simulink model "EthanModel"  (R2019b)
settings: Solver=VariableStepAuto  StartTime=0.0  StopTime=10  RelTol=1e-3
values from neighbouring files (symbols this model uses):
  A = double(round(subs(J_x,   [states, inputs], [trim_state, trim_input])*1000)/1000)    [matlab_init.m]
  A_double = [0 1; 0 0]    [matlab_init.m]
  A_s_double = eval(subs(Ad_double,Ts))    [matlab_init.m]
  A_s_single = eval(subs(Ad_single,Ts))    [matlab_init.m]
  A_single = [0]    [matlab_init.m]
  Aaileron = A(5:8,5:8)    [matlab_init.m]
  Aelevator = A(1:4,1:4)    [matlab_init.m]
  Arudder = A(11:12,11:12)    [matlab_init.m]
  Athrust = A(9:10,9:10)    [matlab_init.m]
  B = B*MotorMix    [matlab_init.m]
  B_double = [0; 1]    [matlab_init.m]
  B_s_double = eval(subs(Bd_double,Ts))    [matlab_init.m]
  B_s_single = eval(subs(Bd_single,Ts))    [matlab_init.m]
  B_single = [1]    [matlab_init.m]
  Baileron = B(5:8,3)    [matlab_init.m]
  Belevator = B(1:4,2)    [matlab_init.m]
  Brudder = B(11:12,4)    [matlab_init.m]
  Bthrust = B(9:10,1)    [matlab_init.m]
  C = double(round(subs(J_y,   [states, inputs], [trim_state, trim_input])*1000)/1000)    [matlab_init.m]
  C_double = [1 0]    [matlab_init.m]
  C_P = 0.041    [matlab_init.m]
  C_rollpitch = rho*prop_dia^4*prop_dist/sqrt(2)*[                 1  -1  -1   1 ;                 1   1  -1  -1 ;                 0   0   0   0 ; ]    [matlab_init.m]
  C_single = [1]    [matlab_init.m]
  C_T = [0.069075;4.95e-05]    [matlab_init.m]
  C_yaw = rho*prop_dia^5/(2*pi)*[                 0   0   0   0 ;                 0   0   0   0 ;                -1   1  -1   1 ; ]    [matlab_init.m]
  Caileron = [0 1 0 0; 0 0 0 1]    [matlab_init.m]
  Celevator = [0 1 0 0; 0 0 0 1]    [matlab_init.m]
  Crudder = [0 1]    [matlab_init.m]
  Cthrust = [ 1 0; 0 0]    [matlab_init.m]
  D = D*MotorMix    [matlab_init.m]
  D_double = [0]    [matlab_init.m]
  D_single = [0]    [matlab_init.m]
  Daileron = [0 ; 0]    [matlab_init.m]
  Delevator = [0 ; 0]    [matlab_init.m]
  Drudder = 0    [matlab_init.m]
  Dthrust = [0 ; D(4,1)]    [matlab_init.m]
  g = [0;0;UAV_mass*9.81]    [matlab_init.m]
  I_flip = eye(12)    [matlab_init.m]
  J = [      Jxx   0   0 ;       0   Jyy  0 ;       0    0  Jzz; ]    [matlab_init.m]
  Jinv = inv(J)    [matlab_init.m]
  L_double = lqe(A_double, G_double, C_double, q_double, r_double, 0)    [matlab_init.m]
  L_single = lqe(A_single, G_single, C_single, q_single, r_single, 0)    [matlab_init.m]
  measurement_noise = 0.1    [matlab_init.m]
  MotorMix = [                 1  1  1 -1 ;                 1  1 -1  1 ;                 1 -1 -1 -1 ;                 1 -1  1  1 ; ]    [matlab_init.m]
  omega_c = 2*pi *20    (= 125.663706144)    [matlab_init.m]
  process_noise = 0.05    [matlab_init.m]
  Prop_H = 2*pi*Jprop*[               0  0  0  0 ;               0  0  0  0 ;               1 -1  1 -1 ; ]    [matlab_init.m]
  q_single = cov(out.In_Out_Data{1}.Values.Data)*10000000000000    [matlab_init.m]
  r_single = cov(out.In_Out_Data{2}.Values.Data)    [matlab_init.m]
  tau2 = 1/(20*pi)    (= 0.0159154943092)    [matlab_init.m]
  Thrust_Sum = rho*prop_dia^4*[                 0   0   0   0 ;                 0   0   0   0 ;                -1  -1  -1  -1 ; ]    [matlab_init.m]
  trim_input = [293,293,293,293]    [matlab_init.m]
  trim_state = [0,0,0,0,0,0,0,0,0,0,0,0]    [matlab_init.m]
  Ts = 0.005    [matlab_init.m]
  UAV_mass = 0.068    [matlab_init.m]
undefined symbols (not defined in the file or in its folder): DiscIntNeverNeededParam, Discrete, Time
libraries: ctrlSharedLib x10, simulink x4, vrlib x3, dspmtrx3 x1
(part 1 of 2)
settings Model: Creator=Chris  LastModifiedBy=ethan

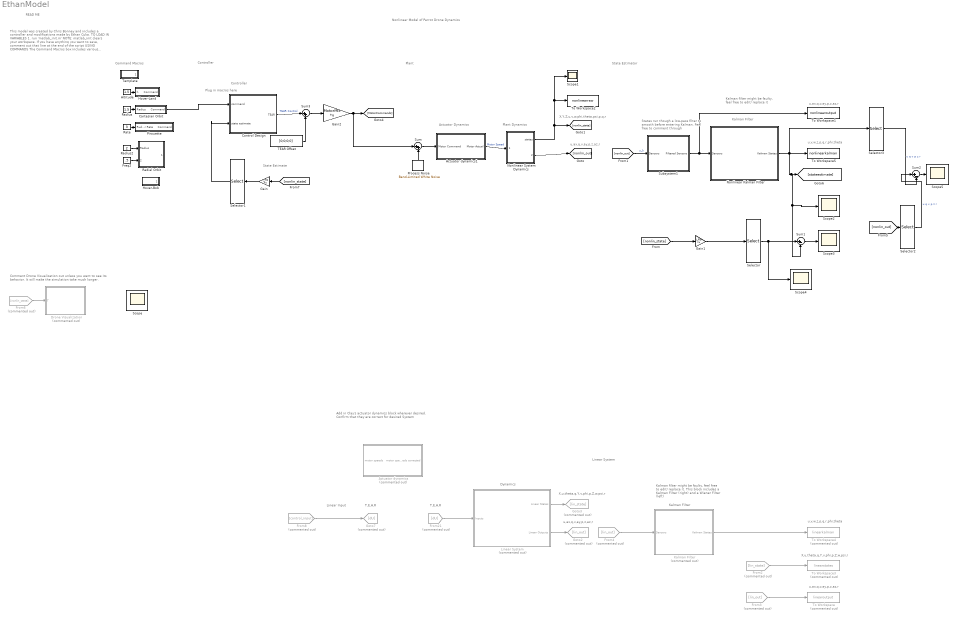
== system EthanModel ==
  note: Plug in macros here
  note: State Estimator
  note: Controller
  note: Command Macros
  note: Add in Clay's actuator dynamics block wherever desired.
      | Confirm that they are correct for desired System
  note: States run though a low-pass filter
      | to smooth before entering Kalman.
      | Feel free to comment through
  note: Kalman filter might be faulty,
      | feel free to edit/ replace it
  note: Comment Drone Visualization out unless you want to see
      | its behavior. It will make the simulation take much longer.
  note: Linear Input
  note: This model was created by Chris Bonney and
      | includes a controller and modifications made
      | by Ethan Cuka.
      |
      |
      | TO LOAD IN VARIABLES
      | 1. run 'matlab_init.m'
      |
      |
      | NOTE: matlab_init clears your workspace.
      | If you have anything you want to save,
      | comment out that line at the end of the script
      |
      |
      | USING COMMANDS
      | The Command Macros box includes various
      | commands to issue to the UAV. To use them,
      | attach their output to the "command" input of
      | the Controller subsystem.
      |
      |
      | READING OUTPUTS
      | most outputs should have a list of variables
      | above them, which are the order they are in
      | for the vector
      |
      |
      | NOISE
      | process and measurement noise blocks are all
      | included in the design, but set to zero power
      | (off); to turn them on go in and adjust their
      | power, there are preset values for noises in
      | kalman_matrices_calculator.m
      |
      |
      | VISUALIZATION
      | 1. the drone visualization block (below) can be
      | uncommented to see the drone fly while
      | running the simulation.
      | 2. I created a scope block (right) that can be
      | copied with preset settings to make viewing
      | data easier
  note: Plant
  note: Kalman Filter
  note: Plant Dynamics
  note: Nonlinear Model of Parrot Drone Dynamics
  note: u,ax,q,v,ay,p,z,az,r
  note: u,v,w,z,p,q,r,phi,theta
  note: Linear System
  note: u,ax,q,v,ay,p,z,az,r
  note: X,u,theta,q,Y,v,phi,p,Z,w,psi,r
  note: u,ax,q,v,ay,p,z,az,r
  note: u,v,w,z,p,q,r,phi,theta
  note: Dynamics
  note: Kalman Filter
  note: Kalman filter might be faulty,
      | feel free to edit/ replace it. This
      | block includes a Kalman Filter (right)
      | and a Wiener Filter (left)
  note: X,Y,Z,u,v,w,phi,theta,psi,p,q,r
  note: u,ax,q,v,ay,p,z,az,r
  note: X,u,theta,q,Y,v,phi,p,Z,w,psi,r
  note: READ ME
  note: T,E,A,R
  note: T,E,A,R
  note: Actuator Dynamics
  note: Controller
  note: State Estimate
  Actuator dynamics : Subsystem  Commented=on
  Actuator dynamics1 : Subsystem
  Altitude : Constant  Value=1.5
  Cartesian Orbit : Subsystem
  Control Design : Subsystem
  Drone Visualization : MATLAB Function  Commented=on  TreatAsAtomicUnit=on
  Freq2 : Constant  Value=.5
  From2 : From  Commented=on  GotoTag=lin_state
  From21 : From  Commented=on  GotoTag=dU
  From3 : From  Commented=on  GotoTag=lin_out
  From4 : From  Commented=on  GotoTag=lin_out
  From6 : From  Commented=on  GotoTag=nonlin_state
  From8 : From  Commented=on  GotoTag=control_input
  Gain : Gain  Gain=I_flip  Multiplication=Matrix(K*u)
  Gain1 : Gain  Gain=I_flip  Multiplication=Matrix(K*u)
  Gain2 : Gain  Gain=MotorMix  Multiplication=Matrix(K*u)
      settings: AttributesFormatString=%<Gain>
  Goto2 : Goto  Commented=on  GotoTag=lin_out
  Goto3 : Goto  Commented=on  GotoTag=lin_state
  Goto7 : Goto  Commented=on  GotoTag=dU
  Hover-Bob : Subsystem
  Hover-Land : Subsystem
  Kalman Filter : Subsystem  Commented=on
  Linear System : Subsystem  Commented=on
  Nonlinear Kalman Filter : Subsystem
  Nonlinear System Dynamics : Subsystem
  Pirouette : Subsystem
  Process Noise : simulink/Sources/Band-Limited White Noise  Cov=process_noise*ones(4,1)*0  Ts=0.05  seed=[1;2;3;4]
  Radial Orbit : Subsystem
  Radius : Constant  Value=1.5
  Radius2 : Constant  Value=2
  Rate : Constant  Value=3
  Scope{,1..5} (6 alike) : Scope
  Selector : Selector  InputPortWidth=12  IndexOptions=Index vector (dialog)  Indices=[4 5 6 3 10 11 12 7 8]  OutputSizes=1
  Selector1 : Selector  InputPortWidth=12  IndexOptions=Index vector (dialog)  Indices=[4 5 6 3 10 11 12 7 8]  OutputSizes=1
  Selector2 : Selector  InputPortWidth=9  IndexOptions=Index vector (dialog)  Indices=[1 3 4 6 7 9]  OutputSizes=1
  Selector3 : Selector  InputPortWidth=9  IndexOptions=Index vector (dialog)  Indices=[1 6 2 5 4 7]  OutputSizes=1
  Subsystem1 : Subsystem
  Sum : Sum  Inputs=|++
  Sum1 : Sum  Inputs=|+-
  Sum2 : Sum  Inputs=|+-
  Sum3 : Sum  Inputs=|++
  TEAR Offset : Constant  Value=[0;0;0;0]
  Template : Subsystem
  To Workspace : ToWorkspace  Commented=on  VariableName=linearoutput  SaveFormat=Timeseries  SampleTime=-1
  To Workspace1 : ToWorkspace  VariableName=nonlinearoutput  SaveFormat=Timeseries  SampleTime=-1
  To Workspace2 : ToWorkspace  VariableName=nonlinearraw  SampleTime=-1
  To Workspace3 : ToWorkspace  Commented=on  VariableName=linearstates  SaveFormat=Timeseries  SampleTime=-1
  To Workspace4 : ToWorkspace  Commented=on  VariableName=linearkalman  SaveFormat=Timeseries  SampleTime=-1
  To Workspace5 : ToWorkspace  VariableName=nonlinearkalman  SaveFormat=Timeseries  SampleTime=-1
  wires:
  From4/1 -> Kalman Filter/1(Sensors)
  From8/1 -> Goto7/1
  From3/1 -> To Workspace/1
  From2/1 -> To Workspace3/1
  Subsystem1/1(Filtered Sensors) -> Nonlinear Kalman Filter/1(Sensors), To Workspace1/1
  Linear System/1(Linear States) -> Goto3/1
  Nonlinear Kalman Filter/1(Kalman States) -> Selector3/1, Scope2/1, Sum1/2, [stateestimate], To Workspace5/1
  From21/1 -> Linear System/1("Inputs ")
  Actuator dynamics1/1(Motor Actual) -> Nonlinear System Dynamics/1(inputs n)  "Motor Speed"
  Nonlinear System Dynamics/1(states) -> Scope1/1, To Workspace2/1, [nonlin_state]
  Linear System/2(Linear Outputs) -> Goto2/1
  [nonlin_out] -> Subsystem1/1(Sensors)  "y_k"
  Nonlinear System Dynamics/2(outputs) -> [nonlin_out]
  Kalman Filter/1(Kalman States) -> To Workspace4/1
  From6/1 -> Drone Visualization/1(T)
  Gain2/1 -> Sum/1, [MotorCommands]
  Sum/1 -> Actuator dynamics1/1(Motor Command)
  Process Noise/1 -> Sum/2
  [nonlin_state] -> Gain1/1
  Sum1/1 -> Scope3/1
  [nonlin_state] -> Gain/1
  Gain/1 -> Selector1/1
  Selector/1 -> Scope4/1, Sum1/1
  Radius/1 -> Cartesian Orbit/1(Radius)
  Altitude/1 -> Hover-Land/1(h)
  Gain1/1 -> Selector/1
  Sum2/1 -> Scope5/1
  Selector2/1 -> Sum2/1  "u q v p z r"
  Selector3/1 -> Sum2/2  "u q v p z r"
  [nonlin_out] -> Selector2/1
  Control Design/1(TEAR) -> Sum3/1  "TEAR Control"
  Sum3/1 -> Gain2/1
  TEAR Offset/1 -> Sum3/2
  Selector1/1 -> Control Design/2(state estimate)
  Rate/1 -> Pirouette/1(Rudder Rate)
  Freq2/1 -> Radial Orbit/2(Frequency)
  Radius2/1 -> Radial Orbit/1("Radius ")
  Cartesian Orbit/1(Command) -> Control Design/1(command)

== system EthanModel/Actuator dynamics ==
  note: Ignoring Gain V/V0 because
      | we can correct for it
  motor speeds : Inport
  30ms delay : TransportDelay  DelayTime=30e-3
  Demux : Demux
  Mux : Mux
  Saturation4 : Saturate  UpperLimit=500  LowerLimit=10
  Sum2 : Sum  Inputs=++|
  Transfer Fcn : TransferFcn  Denominator=[tau2 1]
  Transfer Fcn1 : TransferFcn  Denominator=[tau2 1]
  Transfer Fcn2 : TransferFcn  Denominator=[tau2 1]
  actuator transfer function : TransferFcn  Denominator=[tau2 1]
  speed correction : Constant  Value=trim_input(1)
  motor speeds corrected : Outport
  wires:
  speed correction/1 -> Sum2/1
  Sum2/1 -> Saturation4/1
  Demux/2 -> Transfer Fcn1/1
  30ms delay/1 -> Demux/1
  Demux/4 -> actuator transfer function/1
  Demux/1 -> Transfer Fcn/1
  Demux/3 -> Transfer Fcn2/1
  motor speeds/1 -> 30ms delay/1
  Saturation4/1 -> motor speeds corrected/1
  Transfer Fcn/1 -> Mux/1
  Transfer Fcn1/1 -> Mux/2
  Transfer Fcn2/1 -> Mux/3
  actuator transfer function/1 -> Mux/4
  Mux/1 -> Sum2/2

== system EthanModel/Actuator dynamics1 ==
  note: Ignoring Gain V/V0 because
      | we can correct for it
  Motor Command : Inport
  30ms delay : TransportDelay  DelayTime=30e-3
  Constant2 : Constant  Value=trim_input'  VectorParams1D=off
  Demux : Demux
  Mux : Mux
  Saturation4 : Saturate  UpperLimit=500  LowerLimit=10
  Scope : Scope
  Sum2 : Sum  Inputs=++|
  Transfer Fcn : TransferFcn  Denominator=[tau2 1]
  Transfer Fcn1 : TransferFcn  Denominator=[tau2 1]
  Transfer Fcn2 : TransferFcn  Denominator=[tau2 1]
  actuator transfer function : TransferFcn  Denominator=[tau2 1]
  Motor Actual : Outport
  wires:
  Mux/1 -> Sum2/2
  actuator transfer function/1 -> Mux/4
  Transfer Fcn2/1 -> Mux/3
  Transfer Fcn1/1 -> Mux/2
  Transfer Fcn/1 -> Mux/1
  Saturation4/1 -> Scope/1, Motor Actual/1
  Motor Command/1 -> 30ms delay/1
  Demux/3 -> Transfer Fcn2/1
  Demux/1 -> Transfer Fcn/1
  Demux/4 -> actuator transfer function/1
  30ms delay/1 -> Demux/1
  Demux/2 -> Transfer Fcn1/1
  Sum2/1 -> Saturation4/1
  Constant2/1 -> Sum2/1

== system EthanModel/Cartesian Orbit ==
  note: This command macro causes the drone to orbit by giving it a sinusoidal command to the x and y velocities
  Radius : Inport
  Gain : Gain  Gain=1/(2*pi)
  Mux1 : Mux  Inputs=9
  Product : Product  Inputs=3
  Product1 : Product  Inputs=3
  Sine Wave : Sin  Amplitude=3  Phase=-1  SampleTime=0
  Sine Wave1 : Sin  Amplitude=3  Phase=pi/2-1  SampleTime=0
  Step : Step  SampleTime=0
  Step1 : Step  SampleTime=0
  height1 : Constant  Value=1.5
  p1 : Constant  Value=0
  phi1 : Constant  Value=0
  q1 : Constant  Value=0
  r1 : Constant  Value=0
  theta1 : Constant  Value=0
  w1 : Constant  Value=0
  Command : Outport
  wires:
  Product1/1 -> Mux1/2
  Step1/1 -> Product1/1
  Sine Wave1/1 -> Product1/2
  Step/1 -> Product/2
  Sine Wave/1 -> Product/1
  Product/1 -> Mux1/1
  Mux1/1 -> Command/1
  phi1/1 -> Mux1/9
  q1/1 -> Mux1/6
  height1/1 -> Mux1/4
  w1/1 -> Mux1/3
  theta1/1 -> Mux1/8
  p1/1 -> Mux1/5
  r1/1 -> Mux1/7
  Radius/1 -> Gain/1
  Gain/1 -> Product1/3, Product/3

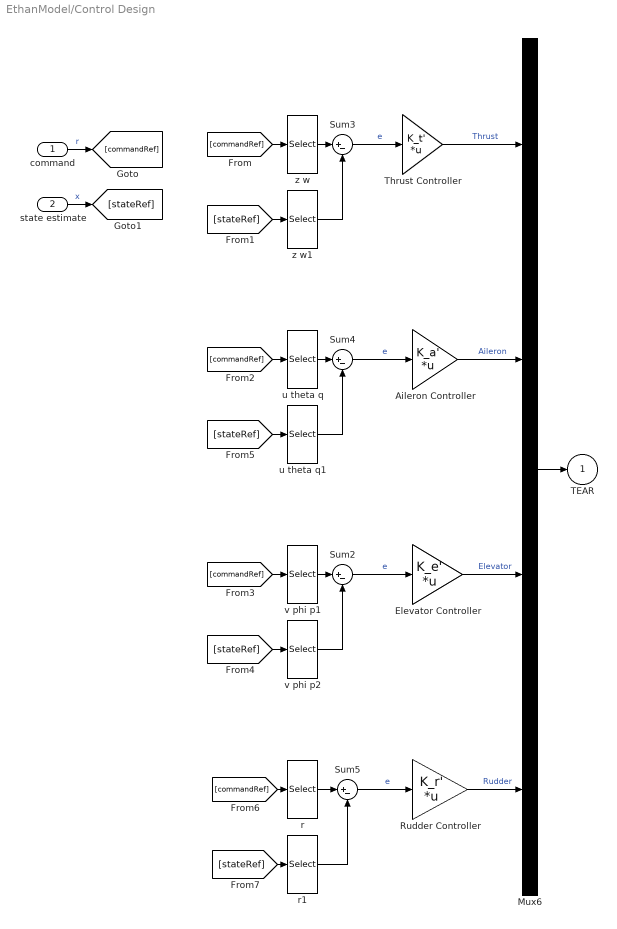
== system EthanModel/Control Design ==
  command : Inport
  state estimate : Inport  Port=2
  Aileron Controller : Gain  Gain=K_a'  Multiplication=Matrix(K*u)
  Elevator Controller : Gain  Gain=K_e'  Multiplication=Matrix(K*u)
  Mux6 : Mux
  Rudder Controller : Gain  Gain=K_r'  Multiplication=Matrix(K*u)
  Sum{2..5} (4 alike) : Sum  Inputs=|+-
  Thrust Controller : Gain  Gain=K_t'  Multiplication=Matrix(K*u)
  r : Selector  InputPortWidth=9  IndexOptions=Index vector (dialog)  Indices=[7]  OutputSizes=1
  r1 : Selector  InputPortWidth=9  IndexOptions=Index vector (dialog)  Indices=[7]  OutputSizes=1
  u theta q : Selector  InputPortWidth=9  IndexOptions=Index vector (dialog)  Indices=[1 9 6]  OutputSizes=1
  u theta q1 : Selector  InputPortWidth=9  IndexOptions=Index vector (dialog)  Indices=[1 9 6]  OutputSizes=1
  v phi p1 : Selector  InputPortWidth=9  IndexOptions=Index vector (dialog)  Indices=[2 8 5]  OutputSizes=1
  v phi p2 : Selector  InputPortWidth=9  IndexOptions=Index vector (dialog)  Indices=[2 8 5]  OutputSizes=1
  z w : Selector  InputPortWidth=9  IndexOptions=Index vector (dialog)  Indices=[4 3]  OutputSizes=1
  z w1 : Selector  InputPortWidth=9  IndexOptions=Index vector (dialog)  Indices=[4 3]  OutputSizes=1
  TEAR : Outport
  wires:
  Mux6/1 -> TEAR/1
  command/1 -> [commandRef]  "r"
  state estimate/1 -> [stateRef]  "x"
  [commandRef] -> z w/1
  [stateRef] -> z w1/1
  z w/1 -> Sum3/1
  z w1/1 -> Sum3/2
  Sum3/1 -> Thrust Controller/1  "e"
  Thrust Controller/1 -> Mux6/1  "Thrust"
  [stateRef] -> v phi p2/1
  v phi p2/1 -> Sum2/2
  [commandRef] -> v phi p1/1
  v phi p1/1 -> Sum2/1
  u theta q/1 -> Sum4/1
  [commandRef] -> u theta q/1
  u theta q1/1 -> Sum4/2
  Sum4/1 -> Aileron Controller/1  "e"
  [stateRef] -> u theta q1/1
  [commandRef] -> r/1
  [stateRef] -> r1/1
  r/1 -> Sum5/1
  r1/1 -> Sum5/2
  Sum2/1 -> Elevator Controller/1  "e"
  Sum5/1 -> Rudder Controller/1  "e"
  Rudder Controller/1 -> Mux6/4  "Rudder"
  Aileron Controller/1 -> Mux6/2  "Aileron"
  Elevator Controller/1 -> Mux6/3  "Elevator"

== system EthanModel/Hover-Bob ==
  note: This command macro causes the drone to hover up and down by commanding the altitude to follow a square wave with DC offset
  Constant : Constant  Value=.5
  Mux : Mux  Inputs=9
  Pulse Generator : DiscretePulseGenerator  PulseType=Time based  Amplitude=1.5  Period=3  PulseWidth=50
  Sum : Sum  Inputs=|++
  p : Constant  Value=0
  phi : Constant  Value=0
  q : Constant  Value=0
  r : Constant  Value=0
  theta : Constant  Value=0
  u : Constant  Value=0
  v : Constant  Value=0
  w : Constant  Value=0
  Command : Outport
  wires:
  r/1 -> Mux/7
  w/1 -> Mux/3
  phi/1 -> Mux/9
  v/1 -> Mux/2
  q/1 -> Mux/6
  u/1 -> Mux/1
  p/1 -> Mux/5
  theta/1 -> Mux/8
  Mux/1 -> Command/1
  Constant/1 -> Sum/2
  Pulse Generator/1 -> Sum/1
  Sum/1 -> Mux/4

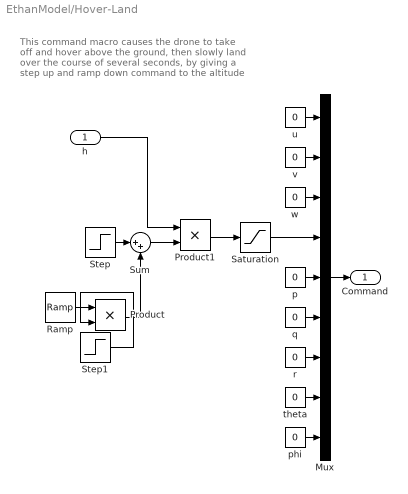
== system EthanModel/Hover-Land ==
  note: This command macro causes the drone to take off and hover above the ground, then slowly land over the course of several seconds, by giving a step up and ramp down command to the altitude
  h : Inport
  Mux : Mux  Inputs=9
  Product : Product
  Product1 : Product
  Ramp : simulink/Sources/Ramp  slope=-.5  start=0  InitialOutput=3.5
  Saturation : Saturate  UpperLimit=100  LowerLimit=0
  Step : Step  SampleTime=0
  Step1 : Step  Time=7  SampleTime=0
  Sum : Sum  Inputs=|++
  p : Constant  Value=0
  phi : Constant  Value=0
  q : Constant  Value=0
  r : Constant  Value=0
  theta : Constant  Value=0
  u : Constant  Value=0
  v : Constant  Value=0
  w : Constant  Value=0
  Command : Outport
  wires:
  Mux/1 -> Command/1
  theta/1 -> Mux/8
  p/1 -> Mux/5
  Product1/1 -> Saturation/1
  u/1 -> Mux/1
  q/1 -> Mux/6
  v/1 -> Mux/2
  phi/1 -> Mux/9
  w/1 -> Mux/3
  r/1 -> Mux/7
  Step/1 -> Sum/1
  Sum/1 -> Product1/2
  Ramp/1 -> Product/1
  Step1/1 -> Product/2
  Product/1 -> Sum/2
  Saturation/1 -> Mux/4
  h/1 -> Product1/1

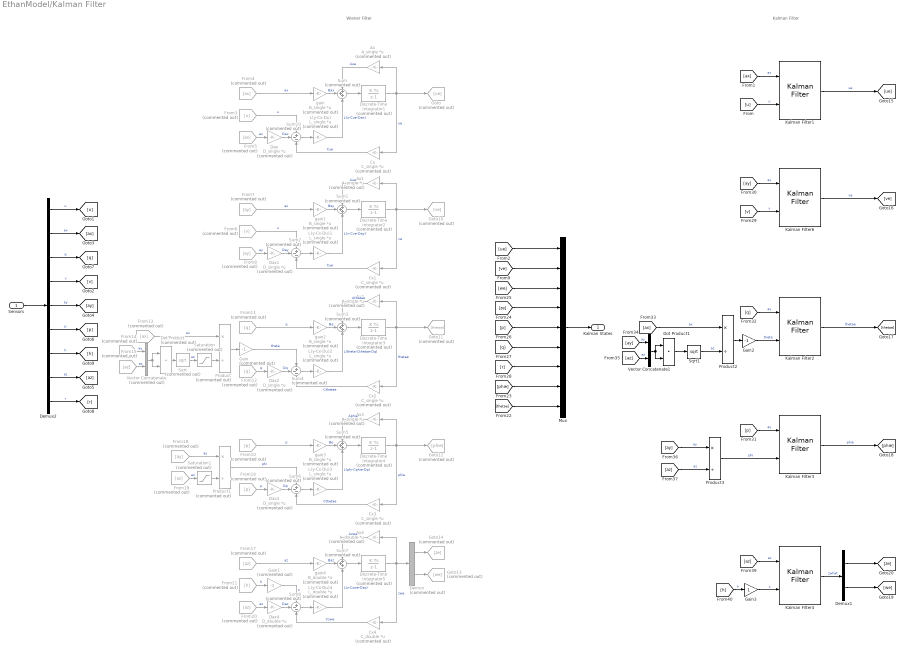
== system EthanModel/Kalman Filter ==
  note: Wiener Filter
  note: Kalman Filter
  Sensors : Inport
  Ax{,1..3} (4 alike) : Gain  Commented=on  Gain=A_single  Multiplication=Matrix(K*u)
      settings: AttributesFormatString=Ax
  Ax4 : Gain  Commented=on  Gain=A_double  Multiplication=Matrix(K*u)
      settings: AttributesFormatString=Ax
  Cx{,1..3} (4 alike) : Gain  Commented=on  Gain=C_single  Multiplication=Matrix(K*u)
      settings: AttributesFormatString=Cx
  Cx4 : Gain  Commented=on  Gain=C_double  Multiplication=Matrix(K*u)
      settings: AttributesFormatString=Cx
  Dax{,1..3} (4 alike) : Gain  Commented=on  Gain=D_single  Multiplication=Matrix(K*u)
      settings: AttributesFormatString=Du
  Dax4 : Gain  Commented=on  Gain=D_double  Multiplication=Matrix(K*u)
      settings: AttributesFormatString=Du
  Demux : Demux  Commented=on  Outputs=2
  Demux1 : Demux  Outputs=2
  Demux2 : Demux  Outputs=9
  Discrete-Time Integrator{1..5} (5 alike) : DiscreteIntegrator  Commented=on  SampleTime=-1  ICPrevOutput=DiscIntNeverNeededParam  ICPrevScaledInput=DiscIntNeverNeededParam
  Dot Product : DotProduct  Commented=on  OutMin=0.0001  InputSameDT=on  OutDataTypeStr=Inherit: Inherit via internal rule
  Dot Product1 : DotProduct  OutMin=0.0001  InputSameDT=on  OutDataTypeStr=Inherit: Inherit via internal rule
  From10 : From  Commented=on  GotoTag=p
  From11 : From  Commented=on  GotoTag=q
  From12 : From  Commented=on  GotoTag=q
  From13 : From  Commented=on  GotoTag=ax
  From{7..8,14,18} (4 alike) : From  Commented=on  GotoTag=ay
  From{15,17,19..20} (4 alike) : From  Commented=on  GotoTag=az
  From16 : From  Commented=on  GotoTag=p
  From21 : From  Commented=on  GotoTag=h
  From3 : From  Commented=on  GotoTag=u
  From4 : From  Commented=on  GotoTag=ax
  From5 : From  Commented=on  GotoTag=ax
  From6 : From  Commented=on  GotoTag=v
  Gain : Gain  Commented=on  Gain=-1
  Gain1 : Gain  Commented=on  Gain=-1
  Gain2 : Gain  Gain=-1
  Gain3 : Gain
  Goto : Goto  Commented=on  GotoTag=ue
  Goto10 : Goto  Commented=on  GotoTag=ve
  Goto11 : Goto  Commented=on  GotoTag=thetae
  Goto12 : Goto  Commented=on  GotoTag=phie
  Goto13 : Goto  Commented=on  GotoTag=we
  Goto14 : Goto  Commented=on  GotoTag=ze
  Kalman Filter{1..3,6} (4 alike) : ctrlSharedLib/Kalman Filter  TimeDomain=Discrete-Time  UseCurrentEstimator=on  ModelSource=Individual A, B, C, D matrices  ModelSourceVariable=ss(0.95,1,1,0,1)  A=A_s_single  B=B_s_single  C=C_single  D=D_single  NumberOfStates=1  NumberOfInputs=1  NumberOfOutputs=1  InitialEstimateSource=Dialog  X0=[0]  P0=10  UseK=off  UseGH=off  NumberOfProcessNoiseInputs=1  G=1  TimeInvariantG=on  H=0  TimeInvariantH=on  Q=[1]*q_single  TimeInvariantQ=on  R=[1]*r_single  TimeInvariantR=on  N=0  TimeInvariantN=on  AddInputPort=on  AddEnablePort=off  OutputEstimatedY=off  OutputP=off  Ts=Ts
      settings: SourceProductBaseCode=CT
  Kalman Filter4 : ctrlSharedLib/Kalman Filter  TimeDomain=Discrete-Time  UseCurrentEstimator=on  ModelSource=Individual A, B, C, D matrices  ModelSourceVariable=ss(0.95,1,1,0,1)  A=A_s_double  B=B_s_double  C=C_double  D=D_double  NumberOfStates=1  NumberOfInputs=1  NumberOfOutputs=1  InitialEstimateSource=Dialog  X0=[0]  P0=10  UseK=off  UseGH=off  NumberOfProcessNoiseInputs=1  G=1  TimeInvariantG=on  H=0  TimeInvariantH=on  Q=[0 0 ; 0 1]*q_single  TimeInvariantQ=on  R=[1]*r_single  TimeInvariantR=on  N=0  TimeInvariantN=on  AddInputPort=on  AddEnablePort=off  OutputEstimatedY=off  OutputP=off  Ts=Ts
      settings: SourceProductBaseCode=CT
  L(y-Cx-Du){,1..3} (4 alike) : Gain  Commented=on  Gain=L_single  Multiplication=Matrix(K*u)
      settings: AttributesFormatString=L(y-Cx-Du)
  L(y-Cx-Du)4 : Gain  Commented=on  Gain=L_double  Multiplication=Matrix(K*u)
      settings: AttributesFormatString=L(y-Cx-Du)
  Mux : Mux  Inputs=9
  Product : Product  Commented=on  Inputs=*/
  Product1 : Product  Commented=on  Inputs=*/
  Product2 : Product  Inputs=*/
  Product3 : Product  Inputs=*/
  Saturation : Saturate  Commented=on  UpperLimit=inf  LowerLimit=0.001
  Saturation1 : Saturate  Commented=on  UpperLimit=inf  LowerLimit=0.001
  Sqrt : Sqrt  Commented=on  SaturateOnIntegerOverflow=on
  Sqrt1 : Sqrt  SaturateOnIntegerOverflow=on
  Sum{,1,3,5,7} (5 alike) : Sum  Commented=on  Inputs=+++
  Sum{2,4,6,8,10} (5 alike) : Sum  Commented=on  Inputs=+--
  Vector Concatenate : Concatenate  Commented=on
  Vector Concatenate1 : Concatenate
  gain{,1..3} (4 alike) : Gain  Commented=on  Gain=B_single  Multiplication=Matrix(K*u)
      settings: AttributesFormatString=Bu
  gain4 : Gain  Commented=on  Gain=B_double  Multiplication=Matrix(K*u)
      settings: AttributesFormatString=Bu
  Kalman States : Outport
  wires:
  Discrete-Time Integrator1/1 -> Goto/1, Cx/1, Ax/1  "ue"
  Sum10/1 -> L(y-Cx-Du)/1
  Ax/1 -> Sum/1  "Aue"
  L(y-Cx-Du)/1 -> Sum/3  "L(u-Cue-Dax)"
  Cx/1 -> Sum10/3  "Cue"
  From4/1 -> gain/1  "ax"
  gain/1 -> Sum/2  "Bax"
  From3/1 -> Sum10/1  "u"
  From5/1 -> Dax/1  "ax"
  Dax/1 -> Sum10/2  "Dax"
  Sum/1 -> Discrete-Time Integrator1/1
  Demux2/1 -> [u]  "u"
  Sensors/1 -> Demux2/1
  Demux2/6 -> [p]  "p"
  Sum1/1 -> Discrete-Time Integrator2/1
  Dax1/1 -> Sum2/2  "Day"
  From8/1 -> Dax1/1  "ay"
  From6/1 -> Sum2/1  "u"
  gain1/1 -> Sum1/2  "Bay"
  From7/1 -> gain1/1  "ax"
  Cx1/1 -> Sum2/3  "Cue"
  L(y-Cx-Du)1/1 -> Sum1/3  "L(v-Cve-Day)"
  Ax1/1 -> Sum1/1  "Aue"
  Sum2/1 -> L(y-Cx-Du)1/1
  Discrete-Time Integrator2/1 -> Ax1/1, Cx1/1, Goto10/1  "ve"
  Discrete-Time Integrator3/1 -> Goto11/1, Cx2/1, Ax2/1  "thetae"
  Sum4/1 -> L(y-Cx-Du)2/1
  Ax2/1 -> Sum3/1  "Athetae"
  L(y-Cx-Du)2/1 -> Sum3/3  "L(theta-Cthetae-Dq)"
  Cx2/1 -> Sum4/3  "Cthetae"
  From11/1 -> gain2/1  "q"
  gain2/1 -> Sum3/2  "Bq"
  Gain/1 -> Sum4/1  "theta"
  From12/1 -> Dax2/1  "q"
  Dax2/1 -> Sum4/2  "Dq"
  Sum3/1 -> Discrete-Time Integrator3/1
  From14/1 -> Vector Concatenate/1  "ay"
  From15/1 -> Vector Concatenate/2  "az"
  Vector Concatenate/1 -> Dot Product/1, Dot Product/2
  Dot Product/1 -> Sqrt/1
  From13/1 -> Product/1  "ax"
  Product/1 -> Gain/1
  From18/1 -> Product1/1  "ay"
  Sum5/1 -> Discrete-Time Integrator4/1
  Dax3/1 -> Sum6/2  "Dp"
  From16/1 -> Dax3/1  "p"
  Product1/1 -> Sum6/1  "phi"
  gain3/1 -> Sum5/2  "Bp"
  From10/1 -> gain3/1  "p"
  Cx3/1 -> Sum6/3  "Cthetae"
  L(y-Cx-Du)3/1 -> Sum5/3  "L(phi-Cphie-Dp)"
  Ax3/1 -> Sum5/1  "Aphie"
  Sum6/1 -> L(y-Cx-Du)3/1
  Discrete-Time Integrator4/1 -> Ax3/1, Cx3/1, Goto12/1  "phie"
  Discrete-Time Integrator5/1 -> Ax4/1, Demux/1, Cx4/1  "zwe"
  Sum8/1 -> L(y-Cx-Du)4/1
  Ax4/1 -> Sum7/1  "Azwe"
  L(y-Cx-Du)4/1 -> Sum7/3  "L(z-Czwe-Daz)"
  Cx4/1 -> Sum8/3  "Czwe"
  From17/1 -> gain4/1  "az"
  gain4/1 -> Sum7/2  "Baz"
  From21/1 -> Gain1/1  "h"
  From20/1 -> Dax4/1  "az"
  Dax4/1 -> Sum8/2  "Daz"
  Sum7/1 -> Discrete-Time Integrator5/1
  Demux/2 -> Goto13/1
  Demux/1 -> Goto14/1
  Gain1/1 -> Sum8/1  "z"
  [ue] -> Mux/1
  [ve] -> Mux/2
  [we] -> Mux/3
  [ze] -> Mux/4
  Mux/1 -> Kalman States/1
  [r] -> Mux/7
  [q] -> Mux/6
  [p] -> Mux/5
  [phie] -> Mux/8
  [thetae] -> Mux/9
  [ax] -> Kalman Filter1/1  "ax"
  [u] -> Kalman Filter1/2  "u"
  [v] -> Kalman Filter6/2  "v"
  [ay] -> Kalman Filter6/1  "ay"
  [q] -> Kalman Filter2/1  "ay"
  Gain2/1 -> Kalman Filter2/2  "theta"
  Sqrt/1 -> Saturation/1  "az"
  Saturation/1 -> Product/2
  From19/1 -> Saturation1/1  "az"
  Saturation1/1 -> Product1/2
  Sqrt1/1 -> Product2/2  "az"
  Product2/1 -> Gain2/1
  [ax] -> Product2/1  "ax"
  Dot Product1/1 -> Sqrt1/1
  Vector Concatenate1/1 -> Dot Product1/2, Dot Product1/1
  [az] -> Vector Concatenate1/2  "az"
  [ay] -> Vector Concatenate1/1  "ay"
  [p] -> Kalman Filter3/1  "ay"
  [az] -> Product3/2  "az"
  Product3/1 -> Kalman Filter3/2  "phi"
  [ay] -> Product3/1  "ay"
  Kalman Filter4/1 -> Demux1/1  "zwhat"
  [az] -> Kalman Filter4/1  "az"
  Gain3/1 -> Kalman Filter4/2  "z"
  Demux1/1 -> [ze]
  Demux1/2 -> [we]
  Kalman Filter3/1 -> [phie]  "phie"
  Kalman Filter2/1 -> [thetae]  "thetae"
  Kalman Filter6/1 -> [ve]  "ve"
  Kalman Filter1/1 -> [ue]  "ue"
  [h] -> Gain3/1  "h"
  Demux2/2 -> [ax]  "ax"
  Demux2/4 -> [v]  "v"
  Demux2/3 -> [q]  "q"
  Demux2/8 -> [az]  "az"
  Demux2/5 -> [ay]  "ay"
  Demux2/7 -> [h]  "h"
  Demux2/9 -> [r]  "r"

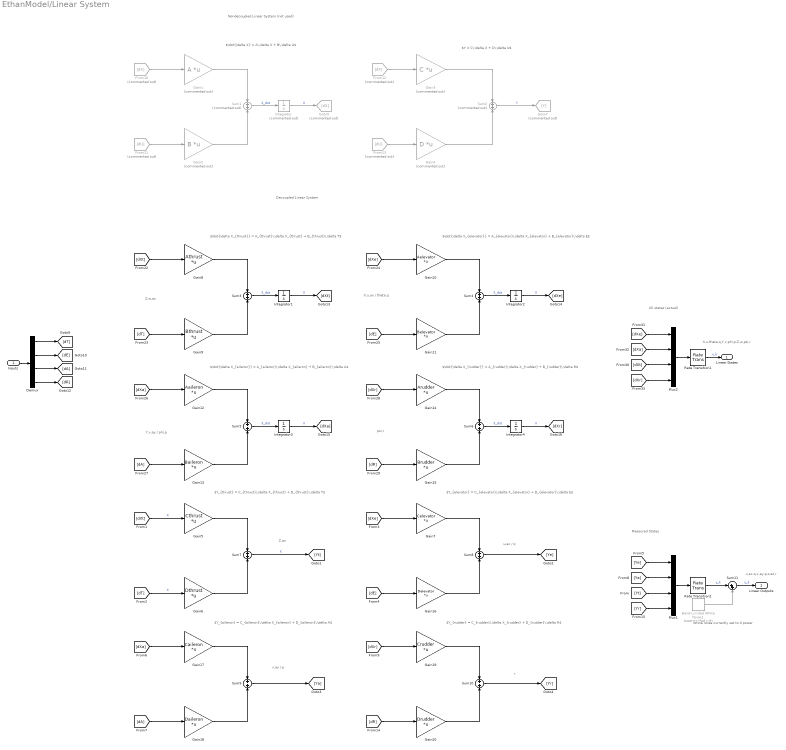
== system EthanModel/Linear System ==
  note: psi,r
  note: Y,v,ay / phi,p
  note: X,u,ax / theta,q
  note: Z,w,az
  note: Decoupled Linear System
  note: $\dot{\delta X} = A\,\delta X + B\,\delta U$
  note: $Y = C\,\delta X + D\,\delta U$
  note: $\dot{\delta X_{thrust}} = A_{thrust}\,\delta X_{thrust} + B_{thrust}\,\delta T$
  note: $\dot{\delta X_{elevator}} = A_{elevator}\,\delta X_{elevator} + B_{elevator}\,\delta E$
  note: $\dot{\delta X_{aileron}} = A_{aileron}\,\delta X_{aileron} + B_{aileron}\,\delta A$
  note: $\dot{\delta X_{rudder}} = A_{rudder}\,\delta X_{rudder} + B_{rudder}\,\delta R$
  note: Z,az
  note: u,ax / q
  note: v,ay / p
  note: r
  note: $Y_{thrust} = C_{thrust}\,\delta X_{thrust} + D_{thrust}\,\delta T$
  note: $Y_{elevator} = C_{elevator}\,\delta X_{elevator} + D_{elevator}\,\delta E$
  note: $Y_{aileron} = C_{aileron}\,\delta X_{aileron} + D_{aileron}\,\delta A$
  note: $Y_{rudder} = C_{rudder}\,\delta X_{rudder} + D_{rudder}\,\delta R$
  note: Nondecoupled Linear System (not used)
  note: All states (actual)
  note: Measured States
  note: u,ax,q,v,ay,p,z,az,r
  note: X,u,theta,q,Y,v,phi,p,Z,w,psi,r
  note: White noise currently set to 0 power
  "Inputs " : Inport
  Band-Limited White Noise1 : simulink/Sources/Band-Limited White Noise  Commented=on  Cov=measurement_noise*ones(9,1)*0  Ts=0.05  seed=[11;12;13;14;15;16;17;18;19]
  Demux : Demux
  From10 : From  Commented=on  GotoTag=dX
  From11 : From  Commented=on  GotoTag=dU
  From12 : From  Commented=on  GotoTag=dX
  From13 : From  Commented=on  GotoTag=dU
  Gain1 : Gain  Commented=on  Gain=A  Multiplication=Matrix(K*u)
  Gain10 : Gain  Gain=Aelevator  Multiplication=Matrix(K*u)
  Gain11 : Gain  Gain=Belevator  Multiplication=Matrix(K*u)
  Gain12 : Gain  Gain=Aaileron  Multiplication=Matrix(K*u)
  Gain13 : Gain  Gain=Baileron  Multiplication=Matrix(K*u)
  Gain14 : Gain  Gain=Arudder  Multiplication=Matrix(K*u)
  Gain15 : Gain  Gain=Brudder  Multiplication=Matrix(K*u)
  Gain16 : Gain  Gain=Delevator  Multiplication=Matrix(K*u)
  Gain17 : Gain  Gain=Caileron  Multiplication=Matrix(K*u)
  Gain18 : Gain  Gain=Daileron  Multiplication=Matrix(K*u)
  Gain19 : Gain  Gain=Crudder  Multiplication=Matrix(K*u)
  Gain2 : Gain  Commented=on  Gain=B  Multiplication=Matrix(K*u)
  Gain20 : Gain  Gain=Drudder  Multiplication=Matrix(K*u)
  Gain3 : Gain  Commented=on  Gain=C  Multiplication=Matrix(K*u)
  Gain4 : Gain  Commented=on  Gain=D  Multiplication=Matrix(K*u)
  Gain5 : Gain  Gain=Cthrust  Multiplication=Matrix(K*u)
  Gain6 : Gain  Gain=Dthrust  Multiplication=Matrix(K*u)
  Gain7 : Gain  Gain=Celevator  Multiplication=Matrix(K*u)
  Gain8 : Gain  Gain=Athrust  Multiplication=Matrix(K*u)
  Gain9 : Gain  Gain=Bthrust  Multiplication=Matrix(K*u)
  Goto5 : Goto  Commented=on  GotoTag=dX
  Goto7 : Goto  Commented=on  GotoTag=Y
  Integrator : Integrator  Commented=on  InitialCondition=trim_state
  Integrator1 : Integrator  InitialCondition=trim_state(9:10)
  Integrator2 : Integrator  InitialCondition=trim_state(1:4)
  Integrator3 : Integrator  InitialCondition=trim_state(5:8)
  Integrator4 : Integrator  InitialCondition=trim_state(11:12)
  Mux1 : Mux
  Mux2 : Mux
  Rate Transition1 : RateTransition  OutPortSampleTime=0.005
  Rate Transition2 : RateTransition  OutPortSampleTime=0.005
  Sum1 : Sum  Commented=on  Inputs=+|+
  Sum{3..10} (8 alike) : Sum  Inputs=+|+
  Sum11 : Sum  Inputs=|++
  Sum2 : Sum  Commented=on  Inputs=+|+
  Linear States : Outport
  Linear Outputs : Outport  Port=2
  wires:
  Gain14/1 -> Sum6/1
  From11/1 -> Gain2/1
  [dXe] -> Gain10/1
  Gain10/1 -> Sum4/1
  Gain2/1 -> Sum1/2
  Gain15/1 -> Sum6/2
  Gain1/1 -> Sum1/1
  Sum5/1 -> Integrator3/1  "X_dot"
  Gain3/1 -> Sum2/1
  Integrator1/1 -> [dXt]  "X"
  From10/1 -> Gain1/1
  Sum1/1 -> Integrator/1  "X_dot"
  Sum2/1 -> Goto7/1  "Y"
  Integrator3/1 -> [dXa]  "X"
  Gain8/1 -> Sum3/1
  [dXt] -> Gain8/1
  Sum3/1 -> Integrator1/1  "X_dot"
  Integrator4/1 -> [dXr]  "X"
  Sum4/1 -> Integrator2/1  "X_dot"
  Gain13/1 -> Sum5/2
  [dXa] -> Gain12/1
  [dXr] -> Gain14/1
  Sum6/1 -> Integrator4/1  "X_dot"
  From13/1 -> Gain4/1
  Gain11/1 -> Sum4/2
  Integrator/1 -> Goto5/1  "X"
  Gain4/1 -> Sum2/2
  Gain12/1 -> Sum5/1
  Integrator2/1 -> [dXe]  "X"
  From12/1 -> Gain3/1
  "Inputs "/1 -> Demux/1
  Demux/3 -> [dA]
  Demux/2 -> [dE]
  Demux/1 -> [dT]
  Demux/4 -> [dR]
  [dXt] -> Mux2/3
  [dXr] -> Mux2/4
  Mux2/1 -> Rate Transition1/1
  [dXe] -> Mux2/1
  [dXa] -> Mux2/2
  Gain6/1 -> Sum7/2
  Gain5/1 -> Sum7/1
  Gain16/1 -> Sum8/2
  [dE] -> Gain16/1
  Gain7/1 -> Sum8/1
  [dXe] -> Gain7/1
  [dA] -> Gain18/1
  Gain17/1 -> Sum9/1
  [dXa] -> Gain17/1
  Gain18/1 -> Sum9/2
  [dXr] -> Gain19/1
  [dR] -> Gain20/1
  Gain20/1 -> Sum10/2
  Gain19/1 -> Sum10/1
  [Ya] -> Mux1/2
  [Ye] -> Mux1/1
  Mux1/1 -> Rate Transition2/1
  [Yr] -> Mux1/4
  [Yt] -> Mux1/3
  [dT] -> Gain9/1
  [dA] -> Gain13/1
  [dR] -> Gain15/1
  [dE] -> Gain11/1
  Sum9/1 -> [Ya]
  Sum10/1 -> [Yr]
  Sum8/1 -> [Ye]
  Sum11/1 -> Linear Outputs/1  "y_k"
  Gain9/1 -> Sum3/2
  [dT] -> Gain6/1  "X"
  [dXt] -> Gain5/1  "X"
  Sum7/1 -> [Yt]  "X"
  Rate Transition1/1 -> Linear States/1  "x_k"
  Band-Limited White Noise1/1 -> Sum11/2
  Rate Transition2/1 -> Sum11/1  "y_k"

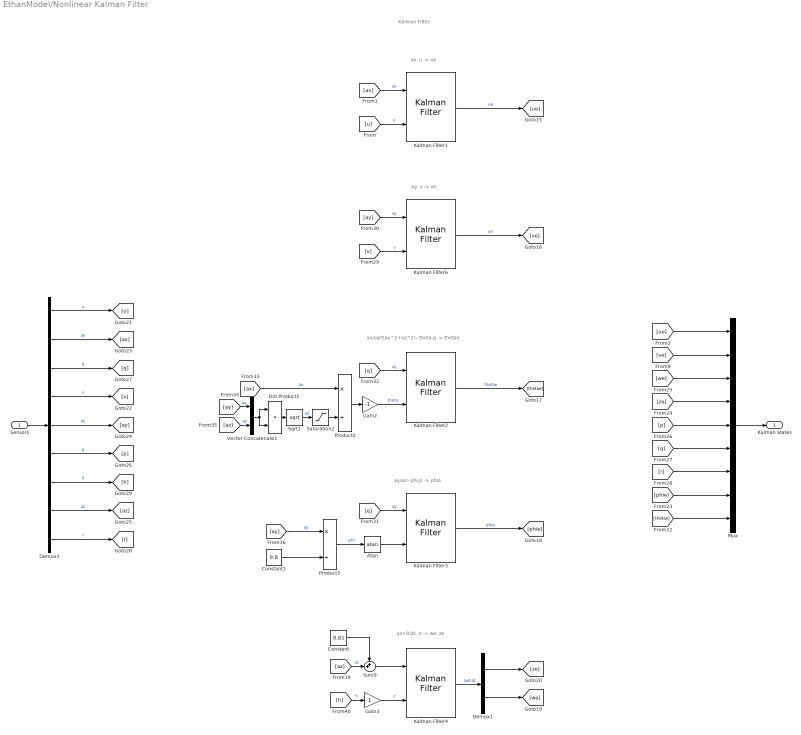
== system EthanModel/Nonlinear Kalman Filter ==
  note: Kalman Filter
  note: ay, v -> ve
  note: ax, u -> ue
  note: ax/sqrt(ay^2+az^2)~theta,q -> thetae
  note: ay/az~phi,p -> phie
  note: az+9.81, z -> we, ze
  Sensors : Inport
  Atan : Trigonometry  Operator=atan
  Constant : Constant  Value=9.81
  Constant1 : Constant  Value=9.8
  Demux1 : Demux  Outputs=2
  Demux3 : Demux  Outputs=9
  Dot Product1 : DotProduct  OutMin=0.0001  InputSameDT=on  OutDataTypeStr=Inherit: Inherit via internal rule
  Gain2 : Gain  Gain=-1
  Gain3 : Gain
  Kalman Filter{1..3,6} (4 alike) : ctrlSharedLib/Kalman Filter  TimeDomain=Discrete-Time  UseCurrentEstimator=on  ModelSource=Individual A, B, C, D matrices  ModelSourceVariable=ss(0.95,1,1,0,1)  A=A_s_single  B=B_s_single  C=C_single  D=D_single  NumberOfStates=1  NumberOfInputs=1  NumberOfOutputs=1  InitialEstimateSource=Dialog  X0=[0]  P0=10  UseK=off  UseGH=off  NumberOfProcessNoiseInputs=1  G=1  TimeInvariantG=on  H=0  TimeInvariantH=on  Q=[1]*q_single  TimeInvariantQ=on  R=[1]*r_single*10000  TimeInvariantR=on  N=0  TimeInvariantN=on  AddInputPort=on  AddEnablePort=off  OutputEstimatedY=off  OutputP=off  Ts=Ts
      settings: SourceProductBaseCode=CT
  Kalman Filter4 : ctrlSharedLib/Kalman Filter  TimeDomain=Discrete-Time  UseCurrentEstimator=on  ModelSource=Individual A, B, C, D matrices  ModelSourceVariable=ss(0.95,1,1,0,1)  A=A_s_double  B=B_s_double  C=C_double  D=D_double  NumberOfStates=1  NumberOfInputs=1  NumberOfOutputs=1  InitialEstimateSource=Dialog  X0=[0]  P0=10  UseK=off  UseGH=off  NumberOfProcessNoiseInputs=1  G=1  TimeInvariantG=on  H=0  TimeInvariantH=on  Q=[0 0; 0 1]*q_single  TimeInvariantQ=on  R=[1]*r_single*10000  TimeInvariantR=on  N=0  TimeInvariantN=on  AddInputPort=on  AddEnablePort=off  OutputEstimatedY=off  OutputP=off  Ts=Ts
      settings: SourceProductBaseCode=CT
  Mux : Mux  Inputs=9
  Product2 : Product  Inputs=*/
  Product3 : Product  Inputs=*/
  Saturation2 : Saturate  UpperLimit=inf  LowerLimit=0.001
  Sqrt1 : Sqrt  SaturateOnIntegerOverflow=on
  Sum9 : Sum  Inputs=++|
  Vector Concatenate1 : Concatenate
  Kalman States : Outport
  wires:
  [h] -> Gain3/1  "h"
  Kalman Filter1/1 -> [ue]  "ue"
  Kalman Filter6/1 -> [ve]  "ve"
  Kalman Filter2/1 -> [thetae]  "thetae"
  Kalman Filter3/1 -> [phie]  "phie"
  Demux1/2 -> [we]
  Demux1/1 -> [ze]
  Gain3/1 -> Kalman Filter4/2  "z"
  Kalman Filter4/1 -> Demux1/1  "zwhat"
  [ay] -> Product3/1  "ay"
  Product3/1 -> Atan/1  "phi"
  [q] -> Kalman Filter3/1  "ay"
  [ay] -> Vector Concatenate1/1  "ay"
  [az] -> Vector Concatenate1/2  "az"
  Vector Concatenate1/1 -> Dot Product1/1, Dot Product1/2
  Dot Product1/1 -> Sqrt1/1
  [ax] -> Product2/1  "ax"
  Product2/1 -> Gain2/1
  Sqrt1/1 -> Saturation2/1  "az"
  Saturation2/1 -> Product2/2
  Gain2/1 -> Kalman Filter2/2  "theta"
  [q] -> Kalman Filter2/1  "ay"
  [ay] -> Kalman Filter6/1  "ay"
  [v] -> Kalman Filter6/2  "v"
  [u] -> Kalman Filter1/2  "u"
  [ax] -> Kalman Filter1/1  "ax"
  [thetae] -> Mux/9
  [phie] -> Mux/8
  [p] -> Mux/5
  [q] -> Mux/6
  [r] -> Mux/7
  Mux/1 -> Kalman States/1
  [ze] -> Mux/4
  [we] -> Mux/3
  [ve] -> Mux/2
  [ue] -> Mux/1
  [az] -> Sum9/2  "az"
  Sum9/1 -> Kalman Filter4/1
  Constant/1 -> Sum9/1
  Demux3/7 -> [h]  "h"
  Demux3/8 -> [az]  "az"
  Demux3/2 -> [ax]  "ax"
  Demux3/1 -> [u]  "u"
  Demux3/4 -> [v]  "v"
  Sensors/1 -> Demux3/1
  Demux3/3 -> [q]  "q"
  Demux3/6 -> [p]  "p"
  Demux3/5 -> [ay]  "ay"
  Demux3/9 -> [r]  "r"
  Atan/1 -> Kalman Filter3/2
  Constant1/1 -> Product3/2

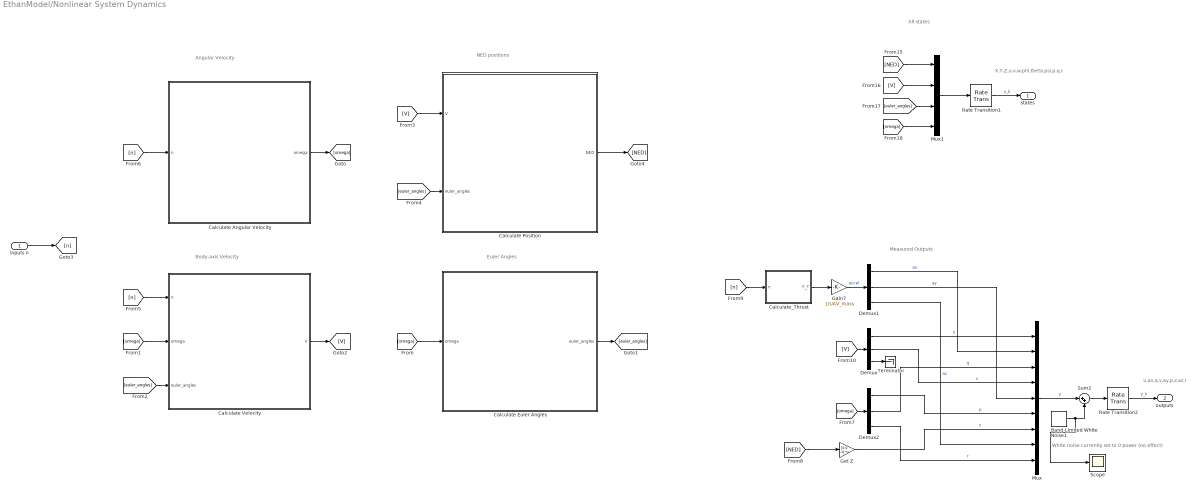
== system EthanModel/Nonlinear System Dynamics ==
  note: White noise currently set to 0 power (no effect)
  note: X,Y,Z,u,v,w,phi,theta,psi,p,q,r
  note: Euler Angles
  note: NED positions
  note: Angular Velocity
  note: Body-axis Velocity
  note: u,ax,q,v,ay,p,z,az,r
  note: All states
  note: Measured Outputs
  inputs n : Inport
  Band-Limited White Noise1 : simulink/Sources/Band-Limited White Noise  Cov=measurement_noise*ones(9,1)*0  Ts=0.05  seed=[11;12;13;14;15;16;17;18;19]
  Calculate Angular Velocity : Subsystem
  Calculate Euler Angles : Subsystem
  Calculate Position : Subsystem
  Calculate Velocity : Subsystem
  Calculate_Thrust : Subsystem
  Demux : Demux  Outputs=3
  Demux1 : Demux  Outputs=3
  Demux2 : Demux  Outputs=3
  Gain7 : Gain  Gain=1/UAV_mass
      settings: AttributesFormatString=%<Gain>
  Get Z : Gain  Gain=[0 0 -1]  Multiplication=Matrix(K*u)
  Mux : Mux  Inputs=9
  Mux1 : Mux
  Rate Transition1 : RateTransition  OutPortSampleTime=0.005
  Rate Transition2 : RateTransition  OutPortSampleTime=0.005
  Scope : Scope
  Sum2 : Sum  Inputs=|++
  Terminator : Terminator
  states : Outport
  outputs : Outport  Port=2
  wires:
  [euler_angles] -> Mux1/3
  [omega] -> Mux1/4
  Calculate Euler Angles/1(euler_angles) -> [euler_angles]
  [V] -> Calculate Position/1("V ")
  [euler_angles] -> Calculate Position/2(euler_angles)
  Calculate Angular Velocity/1(omega) -> [omega]
  [omega] -> Calculate Euler Angles/1(omega)
  Calculate Velocity/1(V) -> [V]
  [V] -> Mux1/2
  [NED] -> Mux1/1
  [euler_angles] -> Calculate Velocity/3(euler_angles)
  [omega] -> Calculate Velocity/2(omega)
  [n] -> Calculate Velocity/1(n)
  Calculate Position/1(NED) -> [NED]
  [n] -> Calculate Angular Velocity/1(n)
  Mux1/1 -> Rate Transition1/1
  inputs n/1 -> [n]
  Demux1/1 -> Mux/2  "ax"
  Demux/1 -> Mux/1  "u"
  Mux/1 -> Sum2/1  "y"
  Demux/3 -> Terminator/1
  Band-Limited White Noise1/1 -> Scope/1, Sum2/2
  [omega] -> Demux2/1
  [NED] -> Get Z/1
  Sum2/1 -> Rate Transition2/1
  Get Z/1 -> Mux/7  "z"
  Demux2/2 -> Mux/3  "q"
  Demux/2 -> Mux/4  "v"
  Demux2/1 -> Mux/6  "p"
  Demux1/2 -> Mux/5  "ay"
  Demux2/3 -> Mux/9  "r"
  [V] -> Demux/1
  Demux1/3 -> Mux/8  "az"
  Gain7/1 -> Demux1/1  "accel"
  Calculate_Thrust/1(F_T) -> Gain7/1
  [n] -> Calculate_Thrust/1(n)
  Rate Transition1/1 -> states/1  "x_k"
  Rate Transition2/1 -> outputs/1  "y_k"

== system EthanModel/Pirouette ==
  note: This command macro rotates the drone in place by giving a constant rudder rate
  Rudder Rate : Inport
  Mux : Mux  Inputs=9
  Product : Product
  Step : Step  SampleTime=0
  height : Constant  Value=1.5
  p : Constant  Value=0
  phi : Constant  Value=0
  q : Constant  Value=0
  theta : Constant  Value=0
  u : Constant  Value=0
  v : Constant  Value=0
  w : Constant  Value=0
  Command : Outport
  wires:
  Mux/1 -> Command/1
  theta/1 -> Mux/8
  p/1 -> Mux/5
  height/1 -> Mux/4
  u/1 -> Mux/1
  q/1 -> Mux/6
  v/1 -> Mux/2
  phi/1 -> Mux/9
  w/1 -> Mux/3
  Step/1 -> Product/2
  Product/1 -> Mux/7
  Rudder Rate/1 -> Product/1

== system EthanModel/Radial Orbit ==
  note: This command macro causes the drone to orbit by giving it a constant tangential velocity and rudder rate
  "Radius " : Inport
  Frequency : Inport  Port=2
  Constant : Constant  Value=0
  Gain : Gain  Gain=2*pi
  Mux1 : Mux  Inputs=9
  Product : Product
  Product1 : Product  Inputs=3
  Step : Step  After=.5  SampleTime=0
  Step1 : Step  After=.5  SampleTime=0
  height1 : Constant  Value=1.5
  p1 : Constant  Value=0
  phi1 : Constant  Value=0
  q1 : Constant  Value=0
  theta1 : Constant  Value=0
  w1 : Constant  Value=0
  Command : Outport
  wires:
  p1/1 -> Mux1/5
  theta1/1 -> Mux1/8
  w1/1 -> Mux1/3
  height1/1 -> Mux1/4
  q1/1 -> Mux1/6
  phi1/1 -> Mux1/9
  Mux1/1 -> Command/1
  Constant/1 -> Mux1/2
  Product/1 -> Product1/3, Mux1/7
  Step/1 -> Product/2
  Gain/1 -> Product/1
  Frequency/1 -> Gain/1
  Product1/1 -> Mux1/1
  "Radius "/1 -> Product1/2
  Step1/1 -> Product1/1

== system EthanModel/Subsystem1 ==
  Sensors : Inport
  Demux3 : Demux  Outputs=9
  Discrete Transfer Fcn{,2..8} (8 alike) : DiscreteTransferFcn  Numerator=[omega_c omega_c]  Denominator=[(omega_c+2/Ts) (omega_c-2/Ts)]  SampleTime=0.005
  Discrete Transfer Fcn1 : DiscreteTransferFcn  Numerator=[omega_c omega_c]  Denominator=[(omega_c+2/Ts) (omega_c-2/Ts)]  InitialStates=.01  SampleTime=0.005
  Mux : Mux  Inputs=9
  Filtered Sensors : Outport
  wires:
  Demux3/6 -> Discrete Transfer Fcn3/1  "p"
  Demux3/5 -> Discrete Transfer Fcn4/1  "ay"
  Demux3/7 -> Discrete Transfer Fcn2/1  "h"
  Demux3/4 -> Discrete Transfer Fcn5/1  "v"
  Demux3/9 -> Discrete Transfer Fcn/1  "r"
  Demux3/8 -> Discrete Transfer Fcn1/1  "az"
  Demux3/2 -> Discrete Transfer Fcn7/1  "ax"
  Sensors/1 -> Demux3/1
  Demux3/3 -> Discrete Transfer Fcn6/1  "q"
  Demux3/1 -> Discrete Transfer Fcn8/1  "u"
  Discrete Transfer Fcn/1 -> Mux/9  "r"
  Discrete Transfer Fcn1/1 -> Mux/8  "az"
  Discrete Transfer Fcn2/1 -> Mux/7  "h"
  Discrete Transfer Fcn3/1 -> Mux/6  "p"
  Discrete Transfer Fcn4/1 -> Mux/5  "ay"
  Discrete Transfer Fcn5/1 -> Mux/4  "v"
  Discrete Transfer Fcn6/1 -> Mux/3  "q"
  Discrete Transfer Fcn7/1 -> Mux/2  "ax"
  Discrete Transfer Fcn8/1 -> Mux/1  "u"
  Mux/1 -> Filtered Sensors/1

== system EthanModel/Template ==
  note: This command macro causes the drone to <do a thing> by <commanding these inputs>
  Mux : Mux  Inputs=9
  height : Constant  Value=1.5
  p : Constant  Value=0
  phi : Constant  Value=0
  q : Constant  Value=0
  r : Constant  Value=0
  theta : Constant  Value=0
  u : Constant  Value=0
  v : Constant  Value=0
  w : Constant  Value=0
  Command : Outport
  wires:
  r/1 -> Mux/7
  w/1 -> Mux/3
  phi/1 -> Mux/9
  v/1 -> Mux/2
  q/1 -> Mux/6
  u/1 -> Mux/1
  height/1 -> Mux/4
  p/1 -> Mux/5
  theta/1 -> Mux/8
  Mux/1 -> Command/1

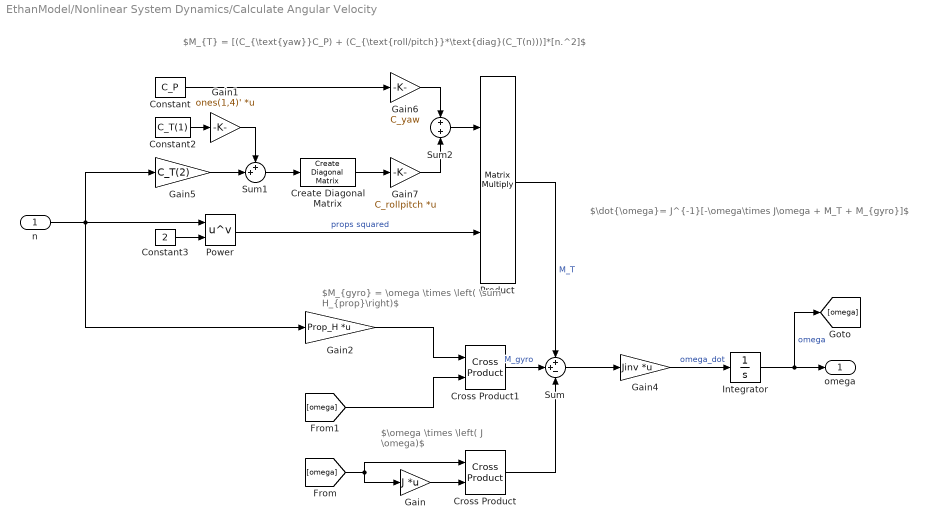
== system EthanModel/Nonlinear System Dynamics/Calculate Angular Velocity ==
  note: $M_{gyro} = \omega \times \left( \sum H_{prop}\right)$
  note: $\dot{\omega}= J^{-1}[-\omega\times J\omega + M_T + M_{gyro}]$
  note: $\omega \times \left( J \omega)$
  note: $M_{T} = [(C_{\text{yaw}}C_P) + (C_{\text{roll/pitch}}*\text{diag}(C_T(n)))]*[n.^2]$
  n : Inport
  Constant : Constant  Value=C_P
  Constant2 : Constant  Value=C_T(1)
  Constant3 : Constant  Value=2
  Create Diagonal Matrix : dspmtrx3/Create Diagonal Matrix
      settings: SourceProductName=DSP System Toolbox  SourceProductBaseCode=DS
  Cross Product : vrlib/Utilities/Cross Product
      settings: SourceProductName=Simulink
  Cross Product1 : vrlib/Utilities/Cross Product
      settings: SourceProductName=Simulink
  Gain : Gain  Gain=J  Multiplication=Matrix(K*u)
  Gain1 : Gain  Gain=ones(1,4)'  Multiplication=Matrix(K*u)
  Gain2 : Gain  Gain=Prop_H  Multiplication=Matrix(K*u)
  Gain4 : Gain  Gain=Jinv  Multiplication=Matrix(K*u)
      settings: AttributesFormatString=%<Gain>
  Gain5 : Gain  Gain=C_T(2)
  Gain6 : Gain  Gain=C_yaw
      settings: AttributesFormatString=%<Gain>
  Gain7 : Gain  Gain=C_rollpitch  Multiplication=Matrix(K*u)
      settings: AttributesFormatString=%<Gain>
  Integrator : Integrator  InitialCondition=[0;0;0]
  Power : Math  Operator=pow  SignedPower=off  SaturateOnIntegerOverflow=on
  Product : Product  Multiplication=Matrix(*)
  Sum : Sum  Inputs=++-
  Sum1 : Sum  Inputs=++|
  Sum2 : Sum  Inputs=+|+
  omega : Outport
  wires:
  Sum/1 -> Gain4/1
  [omega] -> Gain/1, Cross Product/1
  Cross Product/1 -> Sum/3
  [omega] -> Cross Product1/2
  Gain2/1 -> Cross Product1/1
  Cross Product1/1 -> Sum/2  "M_gyro"
  Gain4/1 -> Integrator/1  "omega_dot"
  Gain/1 -> Cross Product/2
  Integrator/1 -> [omega], omega/1  "omega"
  Product/1 -> Sum/1  "M_T"
  Create Diagonal Matrix/1 -> Gain7/1
  Sum2/1 -> Product/1
  Sum1/1 -> Create Diagonal Matrix/1
  Constant/1 -> Gain6/1
  Power/1 -> Product/2  "props squared"
  Gain6/1 -> Sum2/1
  Gain5/1 -> Sum1/2
  Gain7/1 -> Sum2/2
  n/1 -> Gain2/1, Power/1, Gain5/1
  Constant2/1 -> Gain1/1
  Constant3/1 -> Power/2
  Gain1/1 -> Sum1/1

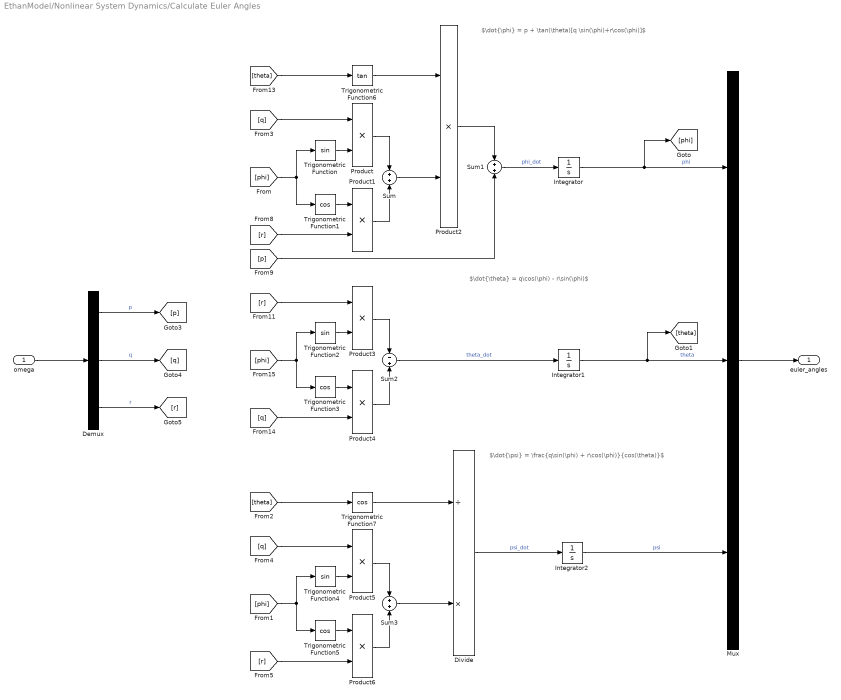
== system EthanModel/Nonlinear System Dynamics/Calculate Euler Angles ==
  note: $\dot{\phi} = p + \tan(\theta)[q \sin(\phi)+r\cos(\phi)]$
  note: $\dot{\theta} = q\cos(\phi) - r\sin(\phi)$
  note: $\dot{\psi} = \frac{q\sin(\phi) + r\cos(\phi)}{cos(\theta)}$
  omega : Inport
  Demux : Demux  Outputs=3
  Divide : Product  Inputs=/*
  Integrator : Integrator  InitialCondition=rand/10
  Integrator1 : Integrator  InitialCondition=rand/10
  Integrator2 : Integrator  InitialCondition=rand/10
  Mux : Mux  Inputs=3
  Product{,1..6} (7 alike) : Product
  Sum : Sum  Inputs=+|+
  Sum1 : Sum  Inputs=+|+
  Sum2 : Sum  Inputs=-|+
  Sum3 : Sum  Inputs=+|+
  Trigonometric Function : Trigonometry
  Trigonometric Function{1,3,5,7} (4 alike) : Trigonometry  Operator=cos
  Trigonometric Function2 : Trigonometry
  Trigonometric Function4 : Trigonometry
  Trigonometric Function6 : Trigonometry  Operator=tan
  euler_angles : Outport
  wires:
  Trigonometric Function7/1 -> Divide/1
  Product1/1 -> Sum/2
  Product6/1 -> Sum3/2
  Trigonometric Function/1 -> Product/2
  Product5/1 -> Sum3/1
  [theta] -> Trigonometric Function7/1
  Trigonometric Function6/1 -> Product2/1
  [r] -> Product6/2
  [theta] -> Trigonometric Function6/1
  Integrator1/1 -> [theta], Mux/2  "theta"
  Trigonometric Function4/1 -> Product5/2
  [q] -> Product4/2
  Demux/3 -> [r]  "r"
  Divide/1 -> Integrator2/1  "psi_dot"
  Integrator2/1 -> Mux/3  "psi"
  [q] -> Product5/1
  Product4/1 -> Sum2/2
  [q] -> Product/1
  [phi] -> Trigonometric Function4/1, Trigonometric Function5/1
  Sum2/1 -> Integrator1/1  "theta_dot"
  Trigonometric Function5/1 -> Product6/1
  Trigonometric Function3/1 -> Product4/1
  [r] -> Product3/1
  Integrator/1 -> [phi], Mux/1  "phi"
  Sum3/1 -> Divide/2
  Product3/1 -> Sum2/1
  [phi] -> Trigonometric Function2/1, Trigonometric Function3/1
  Demux/1 -> [p]  "p"
  Product2/1 -> Sum1/1
  [r] -> Product1/2
  Trigonometric Function1/1 -> Product1/1
  [phi] -> Trigonometric Function1/1, Trigonometric Function/1
  omega/1 -> Demux/1
  Product/1 -> Sum/1
  Demux/2 -> [q]  "q"
  Sum/1 -> Product2/2
  Mux/1 -> euler_angles/1
  Sum1/1 -> Integrator/1  "phi_dot"
  [p] -> Sum1/2
  Trigonometric Function2/1 -> Product3/2

== system EthanModel/Nonlinear System Dynamics/Calculate Position ==
  note: $R(\phi,\theta,\psi)^{-1} = [R(\psi) R(\theta) R(\psi)]^T$
  note: $\dot{NED} = R(\phi,\theta,\psi)^{-1}V$
  "V " : Inport
  euler_angles : Inport  Port=2
  Integrator : Integrator  InitialCondition=[0;0;0]
  Product2 : Product  Multiplication=Matrix(*)
  Rotation_Matrix : Subsystem
  Transpose : Math  Operator=transpose  SignedPower=off  SaturateOnIntegerOverflow=on
  NED : Outport
  wires:
  Product2/1 -> Integrator/1  "NED_dot"
  "V "/1 -> [V]
  Rotation_Matrix/1(Rotation_Matrix) -> Transpose/1  "Rotation_Matrix"
  Transpose/1 -> Product2/1  "Inverse_Rotation_Matrix"
  [V] -> Product2/2
  euler_angles/1 -> Rotation_Matrix/1("euler_angles ")
  Integrator/1 -> NED/1

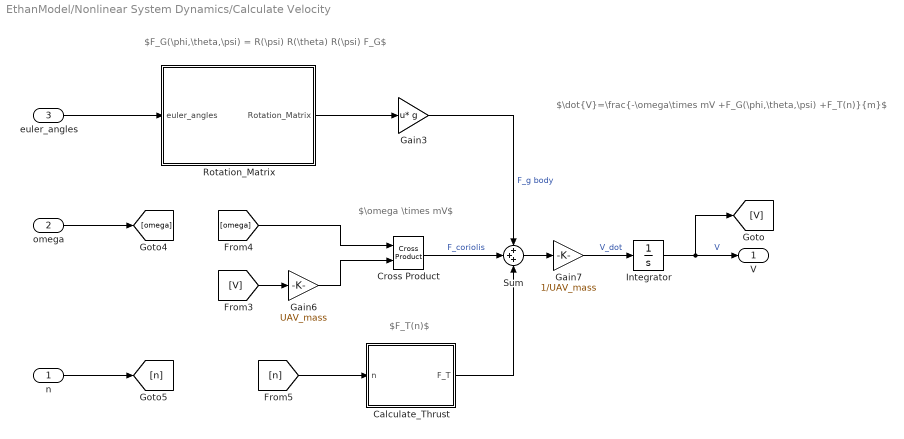
== system EthanModel/Nonlinear System Dynamics/Calculate Velocity ==
  note: $F_G(\phi,\theta,\psi) = R(\psi) R(\theta) R(\psi) F_G$
  note: $\dot{V}=\frac{-\omega\times mV +F_G(\phi,\theta,\psi) +F_T(n)}{m}$
  note: $\omega \times mV$
  note: $F_T(n)$
  n : Inport
  omega : Inport  Port=2
  euler_angles : Inport  Port=3
  Calculate_Thrust : Subsystem
  Cross Product : vrlib/Utilities/Cross Product
      settings: SourceProductName=Simulink
  Gain3 : Gain  Gain=g  Multiplication=Matrix(u*K)
      settings: AttributesFormatString=%<Gain>
  Gain6 : Gain  Gain=UAV_mass
      settings: AttributesFormatString=%<Gain>
  Gain7 : Gain  Gain=1/UAV_mass
      settings: AttributesFormatString=%<Gain>
  Integrator : Integrator  InitialCondition=[0;0;0]
  Rotation_Matrix : Subsystem
  Sum : Sum  Inputs=+++
  V : Outport
  wires:
  [V] -> Gain6/1
  [omega] -> Cross Product/1
  Cross Product/1 -> Sum/2  "F_coriolis"
  Gain3/1 -> Sum/1  "F_g body"
  Gain6/1 -> Cross Product/2
  Sum/1 -> Gain7/1
  Integrator/1 -> V/1, [V]  "V"
  omega/1 -> [omega]
  n/1 -> [n]
  Rotation_Matrix/1(Rotation_Matrix) -> Gain3/1
  euler_angles/1 -> Rotation_Matrix/1("euler_angles ")
  [n] -> Calculate_Thrust/1(n)
  Gain7/1 -> Integrator/1  "V_dot"
  Calculate_Thrust/1(F_T) -> Sum/3

== system EthanModel/Nonlinear System Dynamics/Calculate_Thrust ==
  note: $F_{T} = \sum_{i=1}^4[0;0;C_{T}.*n.^2]$
  n : Inport
  Constant15 : Constant  Value=C_T(1)
  Constant16 : Constant  Value=2
  Gain4 : Gain  Gain=Thrust_Sum  Multiplication=Matrix(K*u)
      settings: AttributesFormatString=%<Gain>
  Gain5 : Gain  Gain=C_T(2)
  Power : Math  Operator=pow  SignedPower=off  SaturateOnIntegerOverflow=on
  Product2 : Product
  Sum1 : Sum  Inputs=++|
  F_T : Outport
  wires:
  Constant15/1 -> Sum1/1
  Gain4/1 -> F_T/1  "F_T"
  n/1 -> Power/1, Gain5/1
  Power/1 -> Product2/2  "props squared"
  Gain5/1 -> Sum1/2
  Sum1/1 -> Product2/1
  Product2/1 -> Gain4/1
  Constant16/1 -> Power/2

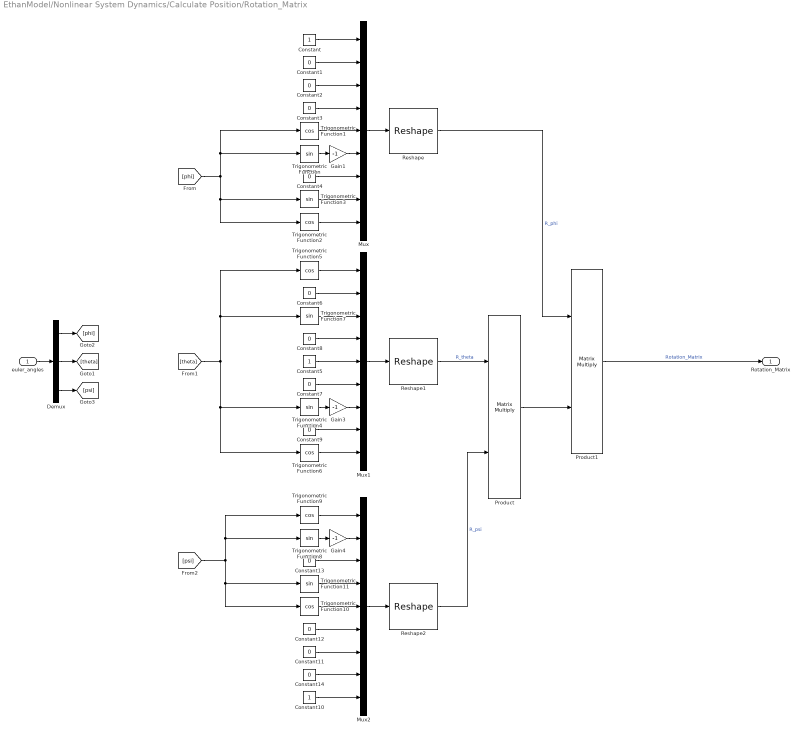
== system EthanModel/Nonlinear System Dynamics/Calculate Position/Rotation_Matrix ==
  "euler_angles " : Inport
  Constant : Constant
  Constant{1..4,6..9,11..14} (12 alike) : Constant  Value=0
  Constant10 : Constant
  Constant5 : Constant
  Demux : Demux  Outputs=3
  Gain1 : Gain  Gain=-1
  Gain3 : Gain  Gain=-1
  Gain4 : Gain  Gain=-1
  Mux : Mux  Inputs=9
  Mux1 : Mux  Inputs=9
  Mux2 : Mux  Inputs=9
  Product : Product  Multiplication=Matrix(*)
  Product1 : Product  Multiplication=Matrix(*)
  Reshape : Reshape  OutputDimensionality=Customize  OutputDimensions=[3,3]
  Reshape1 : Reshape  OutputDimensionality=Customize  OutputDimensions=[3,3]
  Reshape2 : Reshape  OutputDimensionality=Customize  OutputDimensions=[3,3]
  Trigonometric Function{,3..4,7..8,11} (6 alike) : Trigonometry
  Trigonometric Function{1..2,5..6,9..10} (6 alike) : Trigonometry  Operator=cos
  Rotation_Matrix : Outport
  wires:
  Constant9/1 -> Mux1/8
  Constant11/1 -> Mux2/7
  Trigonometric Function1/1 -> Mux/5
  Trigonometric Function3/1 -> Mux/8
  Constant5/1 -> Mux1/5
  Trigonometric Function7/1 -> Mux1/3
  Reshape/1 -> Product1/1  "R_phi"
  Mux1/1 -> Reshape1/1
  Trigonometric Function8/1 -> Gain4/1
  Constant7/1 -> Mux1/6
  Trigonometric Function2/1 -> Mux/9
  [phi] -> Trigonometric Function2/1, Trigonometric Function3/1, Trigonometric Function1/1, Trigonometric Function/1
  Trigonometric Function6/1 -> Mux1/9
  Constant12/1 -> Mux2/6
  Trigonometric Function4/1 -> Gain3/1
  [theta] -> Trigonometric Function7/1, Trigonometric Function5/1, Trigonometric Function4/1, Trigonometric Function6/1
  Reshape2/1 -> Product/2  "R_psi"
  Trigonometric Function/1 -> Gain1/1
  Product/1 -> Product1/2
  Trigonometric Function5/1 -> Mux1/1
  Trigonometric Function9/1 -> Mux2/1
  Mux/1 -> Reshape/1
  Constant/1 -> Mux/1
  Constant3/1 -> Mux/4
  Constant6/1 -> Mux1/2
  Mux2/1 -> Reshape2/1
  Constant2/1 -> Mux/3
  Constant1/1 -> Mux/2
  [psi] -> Trigonometric Function11/1, Trigonometric Function10/1, Trigonometric Function9/1, Trigonometric Function8/1
  Constant8/1 -> Mux1/4
  Constant4/1 -> Mux/7
  Constant13/1 -> Mux2/3
  Trigonometric Function11/1 -> Mux2/4
  Constant10/1 -> Mux2/9
  Reshape1/1 -> Product/1  "R_theta"
  Constant14/1 -> Mux2/8
  Trigonometric Function10/1 -> Mux2/5
  Product1/1 -> Rotation_Matrix/1  "Rotation_Matrix"
  Demux/3 -> [psi]
  Demux/2 -> [theta]
  "euler_angles "/1 -> Demux/1
  Demux/1 -> [phi]
  Gain3/1 -> Mux1/7
  Gain1/1 -> Mux/6
  Gain4/1 -> Mux2/2
